simulink model "example5_9"  (R2016b)
settings: Solver=VariableStepAuto  StartTime=0.0  StopTime=10  RelTol=1e-3
PreLoadFcn:
  | sig=-4:.1:4;
  | sig=exp(sig);
  | V=max(sig);
StopFcn:
  | distor = sum((nocompander-sig).^2)/length(sig);
  | distor2 = sum((withcompander-sig).^2)/length(sig);
  | [distor distor2]
libraries: commsrccod2 x2, dspquant2 x1, dspsrcs4 x1
settings Model: Creator=zhangjin  LastModifiedBy=zhangjin

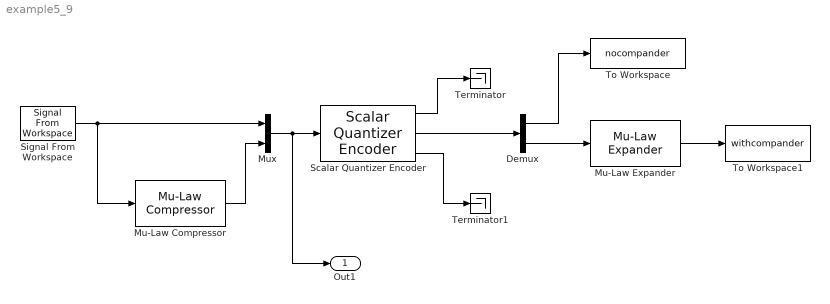
== system example5_9 ==
  Demux : Demux  Outputs=2
  Mu-Law Compressor : commsrccod2/Mu-Law Compressor  mu=255  V=1
  Mu-Law Expander : commsrccod2/Mu-Law Expander  mu=255  V=1
  Mux : Mux  Inputs=2
  Scalar Quantizer Encoder : dspquant2/Scalar Quantizer Encoder  paramSrc=Specify via dialog  partType=Unbounded  BBoundary=[0:floor(V)]  UBoundary=[0:floor(V)]  SearchMethod=Linear  tieBreakRule=Choose the lower index  outQU=on  outQError=on  codebook=[0:ceil(V)]  outStatus=off  invalidin=Error  idtype=int32  roundingMode=Floor  overflowMode=off
  Signal From Workspace : dspsrcs4/Signal From Workspace  X=sig  Ts=1  nsamps=1  OutputAfterFinalValue=Setting to zero  ignoreOrWarnInputAndFrameLengths=off  OutputFrames=off
  Terminator : Terminator
  Terminator1 : Terminator
  To Workspace : ToWorkspace  VariableName=nocompander  SaveFormat=Timeseries  SampleTime=-1
  To Workspace1 : ToWorkspace  VariableName=withcompander  SaveFormat=Timeseries  SampleTime=-1
  Out1 : Outport
  wires:
  Signal From Workspace/1 -> Mu-Law Compressor/1, Mux/1
  Mu-Law Compressor/1 -> Mux/2
  Mux/1 -> Out1/1, Scalar Quantizer Encoder/1
  Scalar Quantizer Encoder/1 -> Terminator/1
  Scalar Quantizer Encoder/3 -> Terminator1/1
  Scalar Quantizer Encoder/2 -> Demux/1
  Demux/1 -> To Workspace/1
  Demux/2 -> Mu-Law Expander/1
  Mu-Law Expander/1 -> To Workspace1/1
